simulink model "etats_paralleles"  (R2020a)
settings: Solver=VariableStepAuto  StartTime=0.0  StopTime=10.0  RelTol=1e-3
settings Model: Creator=ivanl  LastModifiedBy=ivanl

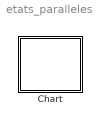
== system etats_paralleles ==
  Chart : Stateflow chart  TreatAsAtomicUnit=on

== stateflow chart etats_paralleles/Chart ==
  state Super_etat_1
    state etat_parallele_1_1 [parallel]
      settings: executionOrder=1
    state etat_parallele_1_2 [parallel]
      settings: executionOrder=2
    state etat_parallele_1_3 [parallel]
      settings: executionOrder=3
    (default) -> etat_parallele_1_1
  state Super_etat_2
    state etat_parallele_2_1 [parallel]
      settings: executionOrder=1
    state etat_parallele_2_2 [parallel]
      settings: executionOrder=2
    state etat_parallele_2_3 [parallel]
      settings: executionOrder=3
    (default) -> etat_parallele_2_1
  (default) -> Super_etat_1
  Super_etat_1 -> Super_etat_2 : [var > 0]
  Super_etat_2 -> Super_etat_1 : [var < 0]
